simulink model "Thingspeak_http"  (R2017b)
settings: Solver=VariableStepAuto  StartTime=0.0  StopTime=10.0  RelTol=1e-3
libraries: mbed_lib x3, mbed_i2c_sensors x2, mbed_spi_several x1, mbed_ethernet x1
settings Model: Creator=oh  LastModifiedBy=oh

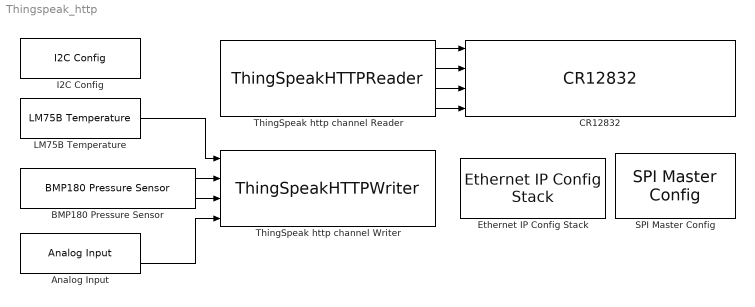
== system Thingspeak_http ==
  Analog Input : mbed_lib/GPIO/Analog Input  PortName=A  PinNumber=0  SampleTime=-1
      settings: SourceProductName=Mbed Target
  BMP180 Pressure Sensor : mbed_i2c_sensors/BMP180 Pressure Sensor  i2cbus=1  SampleTime=-1
      settings: SourceProductName=Mbed Target
  CR12832 : mbed_spi_several/CR12832  TypeOfInputs1={'single'}  NumberOfInputs1=1  Row1='LM75 %f°C'  TypeOfInputs2={'single' 'single'}  NumberOfInputs2=2  Row2='BMP180 %fPa %f°C'  TypeOfInputs3={'single'}  NumberOfInputs3=1  Row3='ADC %fV'  SpiPort=1  CsPort=A  CsPin=0  ResPort=A  ResPin=0  A0Port=A  A0Pin=0  SampleTime=-1
      settings: SourceProductName=Mbed Target
  Ethernet IP Config Stack : mbed_ethernet/Ethernet IP Config Stack  Priority=0  sDHCP=on  DHCP=0  ip_addr=192.168.0.1  sub_mask=255.255.255.0  gateway=0.0.0.0  SerialDebugInfo=off
      settings: SourceProductName=Mbed Target
  I2C Config : mbed_lib/Serial/I2C/I2C Config  Priority=0  I2CPort=1  Freq=100000  SDAPortName=B  SDAPinNumber=9  SCLPortName=B  SCLPinNumber=8
      settings: SourceProductName=Mbed Target
  LM75B Temperature : mbed_i2c_sensors/LM75B Temperature  I2cPort=1  SampleTime=-1
      settings: SourceProductName=Mbed Target
  SPI Master Config : mbed_lib/Serial/SPI/SPI Master Config  Priority=0  SPIPort=1  Freq=100000  Mode=0  Bits=8  MOSIPortNameShow=A  MOSIPortName=0  MOSIPinNumber=7  MISOPortNameShow=A  MISOPortName=0  MISOPinNumber=6  SCLKPortName=A  Parameter13=0  SCLKPinNumber=5
      settings: SourceProductName=Mbed Target
  ThingSpeak http channel Reader : S-Function  Priority=0  FunctionName=ThingSpeakHTTPReader  Parameters=SampleTime, TypeOutputPorts, uint32(BufferSize)  SFunctionDeploymentMode=off  EnableBusSupport=off  mask(Thinkspeak http Reader){channelId='719728', readKey='2KY0I4OUX7V3U5LT', TypeOutputPorts={ 'single' 1 'single' 1 'single' 1 'single' 1 }, field1=Temperatur1, dtype1=single, enable1=on, field2=Temperatur2, dtype2=single, enable2=on, field3=Pressure1, dtype3=single, enable3=on, field4=, dtype4=single, enable4=off, field5=Voltage, dtype5=single, enable5=on, field6=, dtype6=single, enable6=off, field7=, dtype7=single, enable7=off, field8=, dtype8=single, enable8=off, BufferSize=100, SampleTime=15}
      mask prompts: channelId "Channel ID"; readKey "Read Key"; TypeOutputPorts "Type of Outputs"; BufferSize "Buffer Size"; SampleTime "Sample time (-1 for inherited):"
      mask help: Reads upto 8 fields from a channel. Channel names are read from the ThingSpeak channel config. Simulink datatypes has to be adaped manually.
      mask Help: helpview(mbed_getHelpFile('I2CConfig'))
      mask TypeOptions dtype1: single | double | int8 | int16 | int32 | uint8 | uint16 | uint32 | bool
      mask TypeOptions dtype2: single | double | int8 | int16 | int32 | uint8 | uint16 | uint32 | bool
      mask TypeOptions dtype3: single | double | int8 | int16 | int32 | uint8 | uint16 | uint32 | bool
      mask TypeOptions dtype4: single | double | int8 | int16 | int32 | uint8 | uint16 | uint32 | bool
      mask TypeOptions dtype5: single | double | int8 | int16 | int32 | uint8 | uint16 | uint32 | bool
      mask TypeOptions dtype6: single | double | int8 | int16 | int32 | uint8 | uint16 | uint32 | bool
      mask TypeOptions dtype7: single | double | int8 | int16 | int32 | uint8 | uint16 | uint32 | bool
      mask TypeOptions dtype8: single | double | int8 | int16 | int32 | uint8 | uint16 | uint32 | bool
      mask DialogControl Control5 Prompt: load channel config
      mask DialogControl Control5 Callback:
      | maskObj = Simulink.Mask.get(gcb)
      | channelid = maskObj.Parameters(1,1).Value;
      | channelid = channelid(2:size(channelid,2)-1);
      | readkey = maskObj.Parameters(1,2).Value;
      | readkey = readkey(2:size(readkey,2)-1);
      | %[number, fnames] = thinkspeakGetChannelFields('719728', '2KY0I4OUX7V3U5LT');
      | [number, fnames] = thinkspeakGetChannelFields(channelid, readkey);
      | 
      | typeofoutputs = '{';
      | for i=(1:8)
      |   maskObj.Parameters(1,4+(i-1)*3).Value = ' ';
      |   maskObj.Parameters(1,4+(i-1)*3+1).Value = 'single';
      |   maskObj.Parameters(1,4+(i-1)*3+1).Enabled = 'off';
      |   maskObj.Parameters(1,4+(i-1)*3+2).Value = 'off';
      |   maskObj.Parameters(1,4+(i-1)*3+2).Enabled = 'off';
      | end
      | for i=(1:size(number,1))
      |   maskObj.Parameters(1,4+(number(i)-1)*3).Value = char(fnames{i});
      |   maskObj.Parameters(1,4+(number(i)-1)*3+1).Enabled = 'on';
      |   maskObj.Parameters(1,4+(number(i)-1)*3+2).Enabled = 'on';
      |   typeofoutputs = [ typeofoutputs ' ''' maskObj.Parameters(1,4+(number(i)-1)*3+1).Value ''' 1'];
      | end
      | typeofoutputs = [ typeofoutputs ' }'];
      | maskObj.Parameters(1,3).Value = typeofoutputs;
      mask Display:
      | disp(['Thinkspeak\n']);
      | disp(['\nChannel: ' channelId]);
      | pidx=1;
      | if enable1
      |     port_label('output',1,field1);
      |     pidx=pidx+1;
      | end
      | if enable2
      |     port_label('output',pidx,field2);
      |     pidx=pidx+1;
      | end
      | if enable3
      |     port_label('output',pidx,field3);
      |     pidx=pidx+1;
      | end
      | if enable4
      |     port_label('output',pidx,field4);
      |     pidx=pidx+1;
      | end
      | if enable5
      |     port_label('output',pidx,field5);
      |     pidx=pidx+1;
      | end
      | if enable6
      |     port_label('output',pidx,field6);
      |     pidx=pidx+1;
      | end
      | if enable7
      |     port_label('output',pidx,field7);
      |     pidx=pidx+1;
      | end
      | if enable8
      |     port_label('output',pidx,field8);
      |     pidx=pidx+1;
      | end
  ThingSpeak http channel Writer : S-Function  Priority=0  FunctionName=ThingSpeakHTTPWriter  Parameters=SampleTime, TypeInputPorts  SFunctionDeploymentMode=off  EnableBusSupport=off  mask(Thinkspeak http Writer){channelId=719728, writeKey=U48IWT4797KKLW29, TypeInputPorts={ 'single' 1 'single' 1 'single' 1 'single' 1 }, field1=Temperatur1, dtype1=single, enable1=on, field2=Temperatur2, dtype2=single, enable2=on, field3=Pressure1, dtype3=single, enable3=on, field4=, dtype4=single, enable4=off, field5=Voltage, dtype5=single, enable5=on, field6=, dtype6=single, enable6=off, field7=, dtype7=single, enable7=off, field8=, dtype8=single, enable8=off, BufferSize=100, SampleTime=15}
      mask prompts: channelId "Channel ID"; writeKey "Write API Key"; TypeInputPorts "Type of Inputs"; BufferSize "Buffer Size"; SampleTime "Sample time (-1 for inherited):"
      mask help: Writes upto 8 fields to a channel. Channel names are read from the ThingSpeak channel config. Simulink datatypes has to be adaped manually.
      mask Help: helpview(mbed_getHelpFile('I2CConfig'))
      mask TypeOptions dtype1: single | double | int8 | int16 | int32 | uint8 | uint16 | uint32 | bool
      mask TypeOptions dtype2: single | double | int8 | int16 | int32 | uint8 | uint16 | uint32 | bool
      mask TypeOptions dtype3: single | double | int8 | int16 | int32 | uint8 | uint16 | uint32 | bool
      mask TypeOptions dtype4: single | double | int8 | int16 | int32 | uint8 | uint16 | uint32 | bool
      mask TypeOptions dtype5: single | double | int8 | int16 | int32 | uint8 | uint16 | uint32 | bool
      mask TypeOptions dtype6: single | double | int8 | int16 | int32 | uint8 | uint16 | uint32 | bool
      mask TypeOptions dtype7: single | double | int8 | int16 | int32 | uint8 | uint16 | uint32 | bool
      mask TypeOptions dtype8: single | double | int8 | int16 | int32 | uint8 | uint16 | uint32 | bool
      mask DialogControl Control5 Prompt: load channel config
      mask DialogControl Control5 Callback:
      | maskObj = Simulink.Mask.get(gcb);
      | channelid = maskObj.Parameters(1,1).Value;
      | channelid = channelid(2:size(channelid,2)-1);
      | readkey = maskObj.Parameters(1,2).Value;
      | readkey = readkey(2:size(readkey,2)-1);
      | %[number, fnames] = thinkspeakGetChannelFields('719728', '2KY0I4OUX7V3U5LT');
      | [number, fnames] = thinkspeakGetChannelFields(channelid, readkey);
      | 
      | typeofoutputs = '{';
      | for i=(1:8)
      |   maskObj.Parameters(1,4+(i-1)*3).Value = ' ';
      |   maskObj.Parameters(1,4+(i-1)*3+1).Value = 'single';
      |   maskObj.Parameters(1,4+(i-1)*3+1).Enabled = 'off';
      |   maskObj.Parameters(1,4+(i-1)*3+2).Value = 'off';
      |   maskObj.Parameters(1,4+(i-1)*3+2).Enabled = 'off';
      | end
      | for i=(1:size(number,1))
      |   maskObj.Parameters(1,4+(number(i)-1)*3).Value = char(fnames{i});
      |   maskObj.Parameters(1,4+(number(i)-1)*3+1).Enabled = 'on';
      |   maskObj.Parameters(1,4+(number(i)-1)*3+2).Enabled = 'on';
      |   typeofoutputs = [ typeofoutputs ' ''' maskObj.Parameters(1,4+(number(i)-1)*3+1).Value ''' 1'];
      | end
      | typeofoutputs = [ typeofoutputs ' }'];
      | maskObj.Parameters(1,3).Value = typeofoutputs;
      mask Display:
      | disp(['Thinkspeak\n']);
      | disp(['\nChannel: ' channelId]);
      | pidx=1;
      | if enable1
      |     port_label('input',1,field1);
      |     pidx=pidx+1;
      | end
      | if enable2
      |     port_label('input',pidx,field2);
      |     pidx=pidx+1;
      | end
      | if enable3
      |     port_label('input',pidx,field3);
      |     pidx=pidx+1;
      | end
      | if enable4
      |     port_label('input',pidx,field4);
      |     pidx=pidx+1;
      | end
      | if enable5
      |     port_label('input',pidx,field5);
      |     pidx=pidx+1;
      | end
      | if enable6
      |     port_label('input',pidx,field6);
      |     pidx=pidx+1;
      | end
      | if enable7
      |     port_label('input',pidx,field7);
      |     pidx=pidx+1;
      | end
      | if enable8
      |     port_label('input',pidx,field8);
      |     pidx=pidx+1;
      | end
  wires:
  ThingSpeak http channel Reader/2 -> CR12832/2
  ThingSpeak http channel Reader/3 -> CR12832/3
  ThingSpeak http channel Reader/4 -> CR12832/4
  ThingSpeak http channel Reader/1 -> CR12832/1
  Analog Input/2 -> ThingSpeak http channel Writer/4
  BMP180 Pressure Sensor/1 -> ThingSpeak http channel Writer/2
  LM75B Temperature/1 -> ThingSpeak http channel Writer/1
  BMP180 Pressure Sensor/2 -> ThingSpeak http channel Writer/3
